simulink library "AEMS_Standard_Library"  (R2016b)
settings: Solver=ode45  StartTime=0.0  StopTime=10.0  RelTol=1e-3
undefined symbols (not defined in the file or in its folder): BkPY, carto, Cbx_extegr, Cbx_lpegrsys, Cbx_portegr, Cnx_bnk_nr_conf, Cnx_cyl_nr_conf, ConfigManagement, configuration_management, Cxx_dcm_io_tmr_end_xxxx, Cxx_dcm_rt_tmr_end, Cxx_DID_xxxx_IO_max, Cxx_DID_xxxx_IO_min, Cxx_egrhsofs, Cxx_vmaniegi, DEM_DEBOUNCE_FREEZE, DEM_DTR_CTL_INVISIBLE, DEM_DTR_CTL_NORMAL, Dem_DtrId2_XXX, Dem_DtrId3_XXX, Dem_DtrId4_XXX, Dem_DtrId5_XXX, Dem_DtrId6_XXX, Dem_DtrId7_XXX, Dem_DtrId8_XXX, Dem_DtrId9_XXX, Dem_DtrId_XXX, Dem_EnableConditionId2_XXX, Dem_EnableConditionId3_XXX, Dem_EnableConditionId4_XXX, Dem_EnableConditionId5_XXX, Dem_EnableConditionId6_XXX, Dem_EnableConditionId7_XXX, Dem_EnableConditionId8_XXX, Dem_EnableConditionId_XXX, Dem_EventId, Dem_EventId2_XXX, Dem_EventId3_XXX, Dem_EventId4_XXX, Dem_EventId5_XXX, Dem_EventId6_XXX, Dem_EventId7_XXX, Dem_EventId8_XXX, Dem_EventId9_XXX, Dem_EventId_Device_Faulttype, Dem_EventId_XXX, DEM_IUMPR_GENERAL_DENOMINATOR, DEM_OPCYC_IGNITION, Dem_RatioId2_XXX, Dem_RatioId3_XXX, Dem_RatioId4_XXX, Dem_RatioId5_XXX, Dem_RatioId6_XXX, Dem_RatioId7_XXX, Dem_RatioId8_XXX, Dem_RatioId_XXX, Dem_StorageConditionId2_XXX, Dem_StorageConditionId3_XXX, Dem_StorageConditionId4_XXX, Dem_StorageConditionId5_XXX ... (+65)
libraries: AEMS_Standard_Library x477, simulink x2
(part 16 of 39)

== system AEMS_Standard_Library/DCM/AEMS_FXP_TO_FLOAT ==
  fxp : Inport  PortDimensions=1
      settings: AttributesFormatString=<tsample=%<SampleTime>>
  Constant : Constant  Value=Resol  OutDataTypeStr=Inherit: Inherit via back propagation
  Constant1 : Constant  Value=Offset  OutDataTypeStr=Inherit: Inherit via back propagation
  Data Type Conversion : DataTypeConversion
  Product1 : Product  OutDataTypeStr=Inherit: Inherit via back propagation  SaturateOnIntegerOverflow=on  RndMeth=Zero
      settings: AttributesFormatString=SAT = %<SaturateOnIntegerOverflow>
  Sum1 : Sum  OutDataTypeStr=Inherit: Inherit via back propagation  RndMeth=Zero  SaturateOnIntegerOverflow=on  InputSameDT=on
      settings: AttributesFormatString=SAT = %<SaturateOnIntegerOverflow>
  phys : Outport
  wires:
  Data Type Conversion/1 -> Product1/1
  Constant1/1 -> Sum1/2
  Constant/1 -> Product1/2
  Sum1/1 -> phys/1
  fxp/1 -> Data Type Conversion/1
  Product1/1 -> Sum1/1

== system AEMS_Standard_Library/DCM/AEMS_RAM_SET_MAX ==
  input : Inport
      settings: AttributesFormatString=<tsample=%<SampleTime>>
  start : Inport  Port=2  OutDataTypeStr=boolean
      settings: AttributesFormatString=<tsample=%<SampleTime>>
  clear : Inport  Port=3  OutDataTypeStr=boolean
      settings: AttributesFormatString=<tsample=%<SampleTime>>
  MinMax3 : MinMax  Function=max  Inputs=2  SaturateOnIntegerOverflow=on  InputSameDT=on
  Switch1 : Switch  Threshold=0.5  SaturateOnIntegerOverflow=on  InputSameDT=on
      settings: AttributesFormatString=<threshold=%<threshold>>
  Switch5 : Switch  Threshold=0.5  SaturateOnIntegerOverflow=on  InputSameDT=on
      settings: AttributesFormatString=<threshold=%<threshold>>
  Unit Delay : UnitDelay  InitialCondition=initial_value  SampleTime=-1
      settings: AttributesFormatString=<initial=%<X0>>
  imm_const7 : Constant  Value=initial_value  OutDataTypeStr=Inherit: Inherit via back propagation
  max_value : Outport
  wires:
  input/1 -> MinMax3/1  "input"
  Switch1/1 -> Switch5/3
  clear/1 -> Switch5/2  "clear"
  MinMax3/1 -> Switch1/1  "max"
  Unit Delay/1 -> MinMax3/2, Switch1/3
  start/1 -> Switch1/2  "start"
  Switch5/1 -> max_value/1, Unit Delay/1  "max_value"
  imm_const7/1 -> Switch5/1

== system AEMS_Standard_Library/DCM/AEMS_RAM_SET_MIN ==
  input : Inport
      settings: AttributesFormatString=<tsample=%<SampleTime>>
  start : Inport  Port=2  OutDataTypeStr=boolean
      settings: AttributesFormatString=<tsample=%<SampleTime>>
  clear : Inport  Port=3  OutDataTypeStr=boolean
      settings: AttributesFormatString=<tsample=%<SampleTime>>
  MinMax3 : MinMax  Inputs=2  SaturateOnIntegerOverflow=on  InputSameDT=on
  Switch1 : Switch  Threshold=0.5  SaturateOnIntegerOverflow=on  InputSameDT=on
      settings: AttributesFormatString=<threshold=%<threshold>>
  Switch5 : Switch  Threshold=0.5  SaturateOnIntegerOverflow=on  InputSameDT=on
      settings: AttributesFormatString=<threshold=%<threshold>>
  Unit Delay : UnitDelay  InitialCondition=initial_value  SampleTime=-1
      settings: AttributesFormatString=<initial=%<X0>>
  imm_const7 : Constant  Value=initial_value  OutDataTypeStr=Inherit: Inherit via back propagation
  min_value : Outport
  wires:
  input/1 -> MinMax3/1  "input"
  Switch1/1 -> Switch5/3
  clear/1 -> Switch5/2  "clear"
  MinMax3/1 -> Switch1/1  "min"
  Unit Delay/1 -> MinMax3/2, Switch1/3
  start/1 -> Switch1/2  "start"
  Switch5/1 -> min_value/1, Unit Delay/1  "min_value"
  imm_const7/1 -> Switch5/1

== system AEMS_Standard_Library/DCM/AEMS_TO_FXP_WITH_LIMIT ==
  phys_value : Inport
  Data Type Conversion : DataTypeConversion
  Max : Constant  Value=Max  OutDataTypeStr=single
  Min : Constant  Value=Min  OutDataTypeStr=single
  MinMax : MinMax  Inputs=2  OutDataTypeStr=single  RndMeth=Zero  SaturateOnIntegerOverflow=on  InputSameDT=on
  MinMax1 : MinMax  Function=max  Inputs=2  OutDataTypeStr=single  RndMeth=Zero  SaturateOnIntegerOverflow=on  InputSameDT=on
  Offset : Constant  Value=Offset  OutDataTypeStr=single
  OutputDatatype : DataTypeConversion  OutDataTypeStr=int8  SaturateOnIntegerOverflow=on
  Product : Product  Inputs=*/  OutDataTypeStr=single  SaturateOnIntegerOverflow=on  RndMeth=Zero
      settings: AttributesFormatString=SAT = %<SaturateOnIntegerOverflow>
  Resolution : Constant  Value=Resol  OutDataTypeStr=single
  Sum : Sum  Inputs=+-  OutDataTypeStr=single  RndMeth=Zero  SaturateOnIntegerOverflow=on  InputSameDT=on
      settings: AttributesFormatString=SAT = %<SaturateOnIntegerOverflow>
  fxp_value : Outport
  wires:
  Data Type Conversion/1 -> MinMax1/1
  MinMax/1 -> Sum/1
  Resolution/1 -> Product/2
  Min/1 -> MinMax1/2
  OutputDatatype/1 -> fxp_value/1
  Sum/1 -> Product/1
  MinMax1/1 -> MinMax/2
  Max/1 -> MinMax/1
  Offset/1 -> Sum/2
  phys_value/1 -> Data Type Conversion/1
  Product/1 -> OutputDatatype/1

== system AEMS_Standard_Library/DEM/AEMS_DEM_COUNTER_BASED_DEBOUNCE ==
  flag_set : Inport
  conditionfulfilled : Inport  Port=2
  prefailed : Inport  Port=3
  prepassed : Inport  Port=4
  cleardatarequest : Inport  Port=5
  reseteventdebounce : Inport  Port=6
  AEMS_DEM_COUNTER_BASED_DEBOUNCE_D : AEMS_Standard_Library/SUB/AEMS_DEM_COUNTER_BASED_DEBOUNCE_1D  Tag=[LIB]  Description=This subsystem is interface for self diagnosis standard calculated from similar condition and NG judgment.  eventid=Dem_EventId_Device_Faulttype  DemDebounceBehavior1=DEM_DEBOUNCE_FREEZE (0)  DemCounterFailedThreshold=Cnx_dem_fail_thd_Device_Faulttype  DemCounterIncrementStepSize=Cnx_dem_pfail_inc_step_Device_Faulttype  DemCounterJumpUp=Cbx_dem_jmp_up_act_Device_Faulttype  DemCounterJumpUpValue=Cnx_dem_jmp_up_pfail_Device_Faulttype  DemCounterPassedThreshold=Cnx_dem_pass_thd_Device_Faulttype  DemCounterDecrementStepSize=Cnx_dem_ppass_dec_step_Device_Faulttype  DemCounterJumpDown=Cbx_dem_jmp_dwn_act_Device_Faulttype  DemCounterJumpDownValue=Cnx_dem_jmp_dwn_ppass_Device_Faulttype  DemCounterBypassFailure=Cbx_dem_byp_fail_Device_Faulttype
      settings: AttributesFormatString=|
      | %<MaskType>
      | EventId: %<eventid>\nDem Debounce Behavior = %<DemDebounceBehavior1>\nDem Debounce Counter Failed Threshold = %<DemCounterFailedThreshold>\nDem Debounce Counter Increment Step Size = %<DemCounterIncrementStepSize>\nDem Debounce Counter Jump Up = %<DemCounterJumpUp>\nDem Debounce Counter Jump Up Value = %<DemCounterJumpUpValue>\nDem Debounce Counter Passed Threshold = %<DemCounterPassedThreshold>\nDem Debounce Counter Decrement Step Size = %<DemCounterDecrementStepSize>\nDem Debounce Counter Jump Down = %<DemCounterJumpDown>\nDem Debounce Counter Jump Down Value = %<DemCounterJumpDownValue>\nDem Debounce Counter Bypass Failure = %<DemCounterBypassFailure>
  Logical Operator : Logic  Operator=OR  OutDataTypeStr=boolean
  debouncevalue : Outport
  failed : Outport  Port=2
  passed : Outport  Port=3
  wires:
  cleardatarequest/1 -> Logical Operator/1
  reseteventdebounce/1 -> Logical Operator/2
  Logical Operator/1 -> AEMS_DEM_COUNTER_BASED_DEBOUNCE_D/5  "reseteventdebounce"
  flag_set/1 -> AEMS_DEM_COUNTER_BASED_DEBOUNCE_D/1
  conditionfulfilled/1 -> AEMS_DEM_COUNTER_BASED_DEBOUNCE_D/2  "conditionfulfilled"
  prefailed/1 -> AEMS_DEM_COUNTER_BASED_DEBOUNCE_D/3  "prefailed"
  prepassed/1 -> AEMS_DEM_COUNTER_BASED_DEBOUNCE_D/4  "prepassed"
  AEMS_DEM_COUNTER_BASED_DEBOUNCE_D/3 -> passed/1
  AEMS_DEM_COUNTER_BASED_DEBOUNCE_D/2 -> failed/1
  AEMS_DEM_COUNTER_BASED_DEBOUNCE_D/1 -> debouncevalue/1

== system AEMS_Standard_Library/DEM/AEMS_DEM_COUNTER_BASED_DEBOUNCE_THRSHOLD_DYN ==
  flag_set : Inport
  conditionfulfilled : Inport  Port=2
  prefailed : Inport  Port=3
  prepassed : Inport  Port=4
  failedthreshold : Inport  Port=5
  passedthreshold : Inport  Port=6
  cleardatarequest : Inport  Port=7
  reseteventdebounce : Inport  Port=8
  AEMS_DEM_COUNTER_BASED_DEBOUNCE_THRSHOLD_DYN_D : AEMS_Standard_Library/SUB/AEMS_DEM_COUNTER_BASED_DEBOUNCE_THRSHOLD_DYN_1D  Tag=[LIB]  Description=This subsystem is interface for self diagnosis standard calculated from similar condition and NG judgment.  eventid=Dem_EventId_Device_Faulttype  DemDebounceBehavior1=DEM_DEBOUNCE_FREEZE (0)  DemCounterIncrementStepSize=Cnx_dem_pfail_inc_step_Device_Faulttype  DemCounterJumpUp=Cbx_dem_jmp_up_act_Device_Faulttype  DemCounterJumpUpValue=Cnx_dem_jmp_up_pfail_Device_Faulttype  DemCounterDecrementStepSize=Cnx_dem_ppass_dec_step_Device_Faulttype  DemCounterJumpDown=Cbx_dem_jmp_dwn_act_Device_Faulttype  DemCounterJumpDownValue=Cnx_dem_jmp_dwn_ppass_Device_Faulttype  DemCounterBypassFailure=Cbx_dem_byp_fail_Device_Faulttype
      settings: AttributesFormatString=|
      | %<MaskType>\nEventId: %<eventid>
      | Dem Debounce Behavior = %<DemDebounceBehavior1>
      | Dem Debounce Counter Increment Step Size = %<DemCounterIncrementStepSize>
      | Dem Debounce Counter Jump Up = %<DemCounterJumpUp>
      | Dem Debounce Counter Jump Up Value = %<DemCounterJumpUpValue>
      | Dem Debounce Counter Decrement Step Size = %<DemCounterDecrementStepSize>
      | Dem Debounce Counter Jump Down = %<DemCounterJumpDown>
      | Dem Debounce Counter Jump Down Value = %<DemCounterJumpDownValue>
      | Dem Debounce Counter Bypass Failure = %<DemCounterBypassFailure>
  AEMS_SRFLIPFLOP : AEMS_Standard_Library/FLAG/AEMS_SRFLIPFLOP  Tag=[LIB]  init=false
      settings: AttributesFormatString=%<MaskType>\nInitial condition (state of Q): = %<init>
  Data Store Write : DataStoreWrite  DataStoreName=Dem_EventId_Device_Faulttype
  Data Type Conversion : DataTypeConversion
  Logical Operator : Logic  Operator=OR  OutDataTypeStr=boolean
  debouncevalue : Outport
  failed : Outport  Port=2
  passed : Outport  Port=3
  wires:
  cleardatarequest/1 -> Logical Operator/1
  reseteventdebounce/1 -> Logical Operator/2
  Logical Operator/1 -> AEMS_DEM_COUNTER_BASED_DEBOUNCE_THRSHOLD_DYN_D/7  "reseteventdebounce"
  AEMS_DEM_COUNTER_BASED_DEBOUNCE_THRSHOLD_DYN_D/1 -> debouncevalue/1
  AEMS_DEM_COUNTER_BASED_DEBOUNCE_THRSHOLD_DYN_D/2 -> failed/1, AEMS_SRFLIPFLOP/1
  AEMS_DEM_COUNTER_BASED_DEBOUNCE_THRSHOLD_DYN_D/3 -> passed/1, AEMS_SRFLIPFLOP/2
  prepassed/1 -> AEMS_DEM_COUNTER_BASED_DEBOUNCE_THRSHOLD_DYN_D/4  "prepassed"
  prefailed/1 -> AEMS_DEM_COUNTER_BASED_DEBOUNCE_THRSHOLD_DYN_D/3  "prefailed"
  conditionfulfilled/1 -> AEMS_DEM_COUNTER_BASED_DEBOUNCE_THRSHOLD_DYN_D/2  "conditionfulfilled"
  flag_set/1 -> AEMS_DEM_COUNTER_BASED_DEBOUNCE_THRSHOLD_DYN_D/1
  failedthreshold/1 -> AEMS_DEM_COUNTER_BASED_DEBOUNCE_THRSHOLD_DYN_D/5
  passedthreshold/1 -> AEMS_DEM_COUNTER_BASED_DEBOUNCE_THRSHOLD_DYN_D/6
  AEMS_SRFLIPFLOP/1 -> Data Type Conversion/1
  Data Type Conversion/1 -> Data Store Write/1

== system AEMS_Standard_Library/DEM/AEMS_DEM_GET_EVENT_STS ==
  AEMS_DEM_GET_EVENT_STS_D : AEMS_Standard_Library/SUB/AEMS_DEM_GET_EVENT_STS_1D  Tag=[LIB]  EventId=EventId_XXXX  LibType=_DGN  FunctionMode=Dysfunctional
      settings: AttributesFormatString=%<MaskType>\nEventId : = %<EventId>\nDEM Library type : = %<LibType>\nFunction Mode : = %<FunctionMode>
  diag_status_flag : Outport
  wires:
  AEMS_DEM_GET_EVENT_STS_D/1 -> diag_status_flag/1  "diag_status_flag"

== system AEMS_Standard_Library/DEM/AEMS_DEM_GET_INDICATOR_STS ==
  AEMS_DEM_GETINDICATORSTATUS : AEMS_Standard_Library/SUB/AEMS_DEM_GETINDICATORSTATUS  Tag=[LIB]  IndicatorId=0 : IndicatorOff  SimulationMode=0 : Indicator off mode
      settings: AttributesFormatString=|
      | %<MaskType>\nIndicatorId = %<IndicatorId>
      | Simulation Mode = %<SimulationMode>
  IndicatorId_Block : Constant  Value=IndicatorOff  OutDataTypeStr=uint8
  indicator_status : Outport
  wires:
  IndicatorId_Block/1 -> AEMS_DEM_GETINDICATORSTATUS/1
  AEMS_DEM_GETINDICATORSTATUS/1 -> indicator_status/1  "indicator_status"

== system AEMS_Standard_Library/DEM/AEMS_DEM_READ_DATA_PID01 ==
  AEMS_DEM_READDATAOFPID01 : AEMS_Standard_Library/SUB/AEMS_DEM_READDATAOFPID01  Tag=[LIB]
      settings: AttributesFormatString=%<MaskType>
  vpid01 : Outport
  wires:
  AEMS_DEM_READDATAOFPID01/1 -> vpid01/1

== system AEMS_Standard_Library/DEM/AEMS_DEM_REP_IUMPR ==
  denlock_status : Inport
  faultdetect_trigger : Inport  Port=2
  DEM_REP_IUMPR_D : AEMS_Standard_Library/SUB/AEMS_DEM_REP_IUMPR_1D  Tag=[LIB]  RatioId=Dem_RatioId_XXX
      settings: AttributesFormatString=%<MaskType>\nRatioId : = %<RatioId>
  wires:
  faultdetect_trigger/1 -> DEM_REP_IUMPR_D/2  "faultdetect_trigger"
  denlock_status/1 -> DEM_REP_IUMPR_D/1  "denlock_status"

== system AEMS_Standard_Library/DEM/AEMS_DEM_REP_IUMPR_DEN_RELEASE ==
  denlock_status : Inport  OutDataTypeStr=boolean
  DEM_REP_IUMPR_DEN_RELEASE_D : AEMS_Standard_Library/SUB/AEMS_DEM_REP_IUMPR_DEN_RELEASE_1D  Tag=[LIB]  RatioId=Dem_RatioId_XXX
      settings: AttributesFormatString=%<MaskType>\nRatioId : = %<RatioId>
  wires:
  denlock_status/1 -> DEM_REP_IUMPR_DEN_RELEASE_D/1  "denlock_status"

== system AEMS_Standard_Library/DEM/AEMS_DEM_REP_IUMPR_FAULTDETECT ==
  faultdetect_trigger : Inport  OutDataTypeStr=boolean
  DEM_REP_IUMPR_FAULTDETECT_D : AEMS_Standard_Library/SUB/AEMS_DEM_REP_IUMPR_FAULTDETECT_1D  Tag=[LIB]  RatioId=Dem_RatioId_XXX
      settings: AttributesFormatString=%<MaskType>\nRatioId : = %<RatioId>
  wires:
  faultdetect_trigger/1 -> DEM_REP_IUMPR_FAULTDETECT_D/1  "faultdetect_trigger"

== system AEMS_Standard_Library/DEM/AEMS_DEM_SET_DTR ==
  set_flag : Inport  Interpolate=off
  testresult : Inport  Port=2  Interpolate=off
  lowerlimit : Inport  Port=3  Interpolate=off
  upperlimit : Inport  Port=4  Interpolate=off
  ctrl_flag : Inport  Port=5  Interpolate=off
  DEM_SET_DTR_D : AEMS_Standard_Library/SUB/AEMS_DEM_SET_DTR_1DU  Tag=[LIB]  conv_type=0x24  EventId=Dem_DtrId_XXX  resol=1  dlim=0  ulim=65535
      settings: AttributesFormatString=%<MaskType>\nConversion Type : = %<conv_type>\nEventId = %<EventId>\nresolution = %<resol>\nlowerlimit = %<dlim>\nupperlimit = %<ulim>
  wires:
  ctrl_flag/1 -> DEM_SET_DTR_D/5  "ctrl_flag"
  lowerlimit/1 -> DEM_SET_DTR_D/3  "lowerlimit"
  upperlimit/1 -> DEM_SET_DTR_D/4  "upperlimit"
  testresult/1 -> DEM_SET_DTR_D/2  "testresult"
  set_flag/1 -> DEM_SET_DTR_D/1  "set_flag"

== system AEMS_Standard_Library/DEM/AEMS_DEM_SET_ENBL_COND ==
  conditionfulfilled : Inport
  DEM_SET_ENBL_COND_D : AEMS_Standard_Library/SUB/AEMS_DEM_SET_ENBL_COND_1D  Tag=[LIB]  EnCondId=Dem_EnableConditionId_XXX
      settings: AttributesFormatString=%<MaskType>\nEnable Condition Id : = %<EnCondId>
  wires:
  conditionfulfilled/1 -> DEM_SET_ENBL_COND_D/1  "conditionfulfilled"

== system AEMS_Standard_Library/DEM/AEMS_DEM_SET_EVENT_AVL ==
  DEM_SET_EVENT_AVL_D : AEMS_Standard_Library/SUB/AEMS_DEM_SET_EVENT_AVL_1D  Tag=[LIB]  EventId=Dem_EventId  DiagROMFLAG=Diag_ROMFLAG
      settings: AttributesFormatString=%<MaskType>\nEventId = %<EventId>\nDiagROMFLAG = %<DiagROMFLAG>
  dgnsw : Outport
  wires:
  DEM_SET_EVENT_AVL_D/1 -> dgnsw/1

== system AEMS_Standard_Library/DEM/AEMS_DEM_SET_EVENT_DSBL ==
  set_flag : Inport
  DEM_SET_EVENT_DSBL_D : AEMS_Standard_Library/SUB/AEMS_DEM_SET_EVENT_DSBL_1D  Tag=[LIB]  EventId=Dem_EventId_XXX
      settings: AttributesFormatString=%<MaskType>\nEventId : = %<EventId>
  wires:
  set_flag/1 -> DEM_SET_EVENT_DSBL_D/1  "set_flag"

== system AEMS_Standard_Library/DEM/AEMS_DEM_SET_EVENT_STS ==
  diag_set_input_flag : Inport
  AEMS_DEM_SET_EVENT_STS_D : AEMS_Standard_Library/SUB/AEMS_DEM_SET_EVENT_STS_1D  Tag=[LIB]  EventId=Dem_EventId_XXX  LibType=_DGNTRP
      settings: AttributesFormatString=%<MaskType>\nEventId : = %<EventId>\nDEM Library type : = %<LibType>
  wires:
  diag_set_input_flag/1 -> AEMS_DEM_SET_EVENT_STS_D/1  "diag_set_input_flag"

== system AEMS_Standard_Library/DEM/AEMS_DEM_SET_IUMPR_DCOND ==
  condition_status : Inport
  set_flag : Inport  Port=2
  Dem_SetIUMPRDenCondition_Call : Subsystem
  wires:
  set_flag/1 -> Dem_SetIUMPRDenCondition_Call/Enable  "set_flag"
  condition_status/1 -> Dem_SetIUMPRDenCondition_Call/1(condition_status)  "condition_status"

== system AEMS_Standard_Library/DEM/AEMS_DEM_SET_OPCYC_STE ==
  cycle_state : Inport
  set_flag : Inport  Port=2
  AEMS_EDGE_RISING : AEMS_Standard_Library/EDGE/AEMS_EDGE_RISING  Tag=[LIB]  init=false
      settings: AttributesFormatString=|
      | %<MaskType>
      | Initial Value : %<init>
  Dem_SetOperationCycleState_Call : Subsystem
  wires:
  AEMS_EDGE_RISING/1 -> Dem_SetOperationCycleState_Call/Enable  "call"
  cycle_state/1 -> Dem_SetOperationCycleState_Call/1(cycle_state)  "cycle_state"
  set_flag/1 -> AEMS_EDGE_RISING/1  "set_flag"

== system AEMS_Standard_Library/DEM/AEMS_DEM_SET_PFC_CYC_QUALD ==
  set_flag : Inport
  Dem_SetPfcCycleQualified_Call : Subsystem
  wires:
  set_flag/1 -> Dem_SetPfcCycleQualified_Call/Enable  "set_flag"

== system AEMS_Standard_Library/DEM/AEMS_DEM_SET_STORAGE_COND ==
  conditionfulfilled : Inport
  DEM_SET_STORAGE_COND_D : AEMS_Standard_Library/SUB/AEMS_DEM_SET_STORAGE_COND_1D  Tag=[LIB]  StorageCondId=Dem_StorageConditionId_XXX
      settings: AttributesFormatString=%<MaskType>\nStorage Condition Id : = %<StorageCondId>
  wires:
  conditionfulfilled/1 -> DEM_SET_STORAGE_COND_D/1  "conditionfulfilled"

== system AEMS_Standard_Library/DEM/AEMS_DEM_TIME_BASED_DEBOUNCE ==
  flag_set : Inport
  conditionfulfilled : Inport  Port=2  OutDataTypeStr=boolean
  prefailed : Inport  Port=3  OutDataTypeStr=boolean
  prepassed : Inport  Port=4  OutDataTypeStr=boolean
  cleardatarequest : Inport  Port=5  OutDataTypeStr=boolean
  reseteventdebounce : Inport  Port=6  OutDataTypeStr=boolean
  AEMS_DEM_TIME_BASED_DEBOUNCE_D : AEMS_Standard_Library/SUB/AEMS_DEM_TIME_BASED_DEBOUNCE_1D  Tag=[LIB]  Description=This subsystem is interface for self diagnosis standard calculated from similar condition and NG judgment.  eventid=Dem_EventId_Device_Faulttype  DemDebounceBehavior1=DEM_DEBOUNCE_FREEZE (0)  DemDebounceTimeFailedThreshold=Cxx_dem_fail_thd_Device_Faulttype  DemDebounceTimePassedThreshold=Cxx_dem_pass_thd_Device_Faulttype  DemTimeBypassFailure=Cbx_dem_byp_fail_Device_Faulttype  Sample_Time=0.01
      settings: AttributesFormatString=|
      | %<MaskType>
      | EventId: %<eventid>\nDem Debounce Behavior = %<DemDebounceBehavior1>\nDem Debounce Time Failed Threshold = %<DemDebounceTimeFailedThreshold>\nDem Debounce Time Passed Threshold = %<DemDebounceTimePassedThreshold>\nDem Debounce Time Bypass Failure = %<DemTimeBypassFailure>\nSample_Time = %<Sample_Time>
  AEMS_SRFLIPFLOP : AEMS_Standard_Library/FLAG/AEMS_SRFLIPFLOP  Tag=[LIB]  init=false
      settings: AttributesFormatString=%<MaskType>\nInitial condition (state of Q): = %<init>
  Data Store Write : DataStoreWrite  DataStoreName=Dem_EventId_Device_Faulttype
  Data Type Conversion : DataTypeConversion
  Logical Operator : Logic  Operator=OR  OutDataTypeStr=boolean
  debouncevalue_for_failed : Outport
  debouncevalue_for_passed : Outport  Port=2
  failed : Outport  Port=3
  passed : Outport  Port=4
  wires:
  AEMS_DEM_TIME_BASED_DEBOUNCE_D/1 -> debouncevalue_for_failed/1
  AEMS_DEM_TIME_BASED_DEBOUNCE_D/2 -> debouncevalue_for_passed/1
  AEMS_DEM_TIME_BASED_DEBOUNCE_D/3 -> failed/1, AEMS_SRFLIPFLOP/1
  AEMS_DEM_TIME_BASED_DEBOUNCE_D/4 -> passed/1, AEMS_SRFLIPFLOP/2
  prepassed/1 -> AEMS_DEM_TIME_BASED_DEBOUNCE_D/4  "prepassed"
  prefailed/1 -> AEMS_DEM_TIME_BASED_DEBOUNCE_D/3  "prefailed"
  conditionfulfilled/1 -> AEMS_DEM_TIME_BASED_DEBOUNCE_D/2  "conditionfulfilled"
  flag_set/1 -> AEMS_DEM_TIME_BASED_DEBOUNCE_D/1
  Logical Operator/1 -> AEMS_DEM_TIME_BASED_DEBOUNCE_D/5  "reseteventdebounce"
  reseteventdebounce/1 -> Logical Operator/2
  cleardatarequest/1 -> Logical Operator/1
  AEMS_SRFLIPFLOP/1 -> Data Type Conversion/1
  Data Type Conversion/1 -> Data Store Write/1

== system AEMS_Standard_Library/DEM/AEMS_DEM_TIME_BASED_DEBOUNCE_THRSHOLD_DYN ==
  note: prepassed
  flag_set : Inport
  conditionfulfilled : Inport  Port=2  OutDataTypeStr=boolean
  prefailed : Inport  Port=3  OutDataTypeStr=boolean
  prepassed : Inport  Port=4  OutDataTypeStr=boolean
  cleardatarequest : Inport  Port=5  OutDataTypeStr=boolean
  reseteventdebounce : Inport  Port=6  OutDataTypeStr=boolean
  failedthreshold : Inport  Port=7
  passedthreshold : Inport  Port=8
  AEMS_DEM_TIME_BASED_DEBOUNCE_THRSHOLD_DYN_D : AEMS_Standard_Library/SUB/AEMS_DEM_TIME_BASED_DEBOUNCE_THRSHOLD_DYN_1D  Tag=[LIB]  Description=This subsystem is interface for self diagnosis standard calculated from similar condition and NG judgment.  eventid=Dem_EventId_Device_Faulttype  DemDebounceBehavior1=DEM_DEBOUNCE_FREEZE (0)  DemTimeBypassFailure=Cbx_dem_byp_fail_Device_Faulttype  Sample_Time=0.01
      settings: AttributesFormatString=|
      | %<MaskType>
      | EventId: %<eventid>\nDem Debounce Behavior = %<DemDebounceBehavior1>\nDem Debounce Time Bypass Failure = %<DemTimeBypassFailure>\nSample_Time = %<Sample_Time>
  Logical Operator : Logic  Operator=OR  OutDataTypeStr=boolean
  debouncevalue_for_failed : Outport
  debouncevalue_for_passed : Outport  Port=2
  failed : Outport  Port=3
  passed : Outport  Port=4
  wires:
  passedthreshold/1 -> AEMS_DEM_TIME_BASED_DEBOUNCE_THRSHOLD_DYN_D/7  "passedthreshold"
  failedthreshold/1 -> AEMS_DEM_TIME_BASED_DEBOUNCE_THRSHOLD_DYN_D/6  "failedthreshold"
  prefailed/1 -> AEMS_DEM_TIME_BASED_DEBOUNCE_THRSHOLD_DYN_D/3  "prefailed"
  flag_set/1 -> AEMS_DEM_TIME_BASED_DEBOUNCE_THRSHOLD_DYN_D/1
  conditionfulfilled/1 -> AEMS_DEM_TIME_BASED_DEBOUNCE_THRSHOLD_DYN_D/2  "conditionfulfilled"
  prepassed/1 -> AEMS_DEM_TIME_BASED_DEBOUNCE_THRSHOLD_DYN_D/4
  Logical Operator/1 -> AEMS_DEM_TIME_BASED_DEBOUNCE_THRSHOLD_DYN_D/5  "reseteventdebounce"
  AEMS_DEM_TIME_BASED_DEBOUNCE_THRSHOLD_DYN_D/4 -> passed/1
  AEMS_DEM_TIME_BASED_DEBOUNCE_THRSHOLD_DYN_D/3 -> failed/1
  AEMS_DEM_TIME_BASED_DEBOUNCE_THRSHOLD_DYN_D/2 -> debouncevalue_for_passed/1
  AEMS_DEM_TIME_BASED_DEBOUNCE_THRSHOLD_DYN_D/1 -> debouncevalue_for_failed/1
  reseteventdebounce/1 -> Logical Operator/2
  cleardatarequest/1 -> Logical Operator/1

== system AEMS_Standard_Library/DEM/AEMS_FIM_GETFUNCTIONINHIBITION ==
  AEMS_FIM_GET_FUNC_PMT_D : AEMS_Standard_Library/SUB/AEMS_FIM_GET_FUNC_PMT_1D  Tag=[LIB]  FID=Fim_fid_xxxx  FunctionMode=Functional
      settings: AttributesFormatString=%<MaskType>\nFunction Mode = %<FunctionMode>\nDowngraded mode short name : = %<FID>
  InhibitionStatus : Outport
  wires:
  AEMS_FIM_GET_FUNC_PMT_D/1 -> InhibitionStatus/1  "InhibitionStatus"

== system AEMS_Standard_Library/DISCONTINUITIES/AEMS_DEADZONE ==
  input_signal : Inport
  start_end_zone : Inport  Port=2
  end_dead_zone : Inport  Port=3
  Constant1 : Constant  Value=mf  OutDataTypeStr=Inherit: Inherit via back propagation
  Product : Product  OutDataTypeStr=Inherit: Inherit via back propagation  RndMeth=Zero
  RelationalOperator2 : RelationalOperator  Operator=>  OutDataTypeStr=boolean  RndMeth=Nearest  InputSameDT=on
  RelationalOperator3 : RelationalOperator  Operator=<  OutDataTypeStr=boolean  RndMeth=Nearest  InputSameDT=on
  Sum{,1..3} (4 alike) : Sum  Inputs=+-  OutDataTypeStr=Inherit: Inherit via back propagation  RndMeth=Zero  InputSameDT=on
  Switch1 : Switch  Criteria=u2 ~= 0  RndMeth=Zero  SaturateOnIntegerOverflow=on  InputSameDT=on
      settings: AttributesFormatString=Criteria=%<Criteria>
  Switch4 : Switch  Criteria=u2 ~= 0  RndMeth=Zero  SaturateOnIntegerOverflow=on  InputSameDT=on
      settings: AttributesFormatString=Criteria=%<Criteria>
  UnitDelay1 : UnitDelay  SampleTime=-1
      settings: AttributesFormatString=<initial=%<InitialCondition>>
  dead_zone : Outport
  wires:
  start_end_zone/1 -> Sum/2, RelationalOperator2/1
  Switch4/1 -> UnitDelay1/1, dead_zone/1
  RelationalOperator3/1 -> Switch1/2
  RelationalOperator2/1 -> Switch4/2
  Sum3/1 -> Switch1/1
  Switch1/1 -> Switch4/3
  input_signal/1 -> Sum/1, Sum2/1, Sum3/1, Sum1/1
  Sum/1 -> Switch4/1
  end_dead_zone/1 -> RelationalOperator3/1, Sum3/2
  Product/1 -> Switch1/3, Sum1/2, Sum2/2
  UnitDelay1/1 -> Product/1
  Constant1/1 -> Product/2
  Sum1/1 -> RelationalOperator2/2
  Sum2/1 -> RelationalOperator3/2

== system AEMS_Standard_Library/DISCONTINUITIES/AEMS_ENUMERATION_SWITCH ==
  Control_Input : Inport
  Dataport1 : Inport  Port=2
  Dataport2 : Inport  Port=3
  Dataport3 : Inport  Port=4
  MultiportSwitch : MultiPortSwitch  DataPortOrder=Specify indices  Inputs=2  DataPortIndices={[Nnx_aaa_stt,Nnx_bbb_stt],Nnx_ccc_stt,Nnx_ddd_stt}  DiagnosticForDefault=None
  Out : Outport
  wires:
  Dataport2/1 -> MultiportSwitch/3
  Dataport1/1 -> MultiportSwitch/2
  MultiportSwitch/1 -> Out/1
  Control_Input/1 -> MultiportSwitch/1
  Dataport3/1 -> MultiportSwitch/4

== system AEMS_Standard_Library/DISCONTINUITIES/AEMS_MULTI_PORT_TIME_SWITCH ==
  Vxx_swi_t : Inport  Tag=AM,In,0,1,Name,C;CMP,Port,PortWidth,SampleTime;
  Vsx_sel : Inport  Tag=AM,In,0,1,Name,C;CMP,Port,PortWidth,SampleTime;  Port=2
  Vxx_in1 : Inport  Tag=AM,In,0,1,Name,C;CMP,Port,PortWidth,SampleTime;  Port=3
  Vxx_in2 : Inport  Tag=AM,In,0,1,Name,C;CMP,Port,PortWidth,SampleTime;  Port=4
  Vxx_in3 : Inport  Tag=AM,In,0,1,Name,C;CMP,Port,PortWidth,SampleTime;  Port=5
  Vxx_in4 : Inport  Tag=AM,In,0,1,Name,C;CMP,Port,PortWidth,SampleTime;  Port=6
  Vxx_in5 : Inport  Tag=AM,In,0,1,Name,C;CMP,Port,PortWidth,SampleTime;  Port=7
  Vxx_in6 : Inport  Tag=AM,In,0,1,Name,C;CMP,Port,PortWidth,SampleTime;  Port=8
  Vxx_in7 : Inport  Tag=AM,In,0,1,Name,C;CMP,Port,PortWidth,SampleTime;  Port=9
  Vxx_in8 : Inport  Tag=AM,In,0,1,Name,C;CMP,Port,PortWidth,SampleTime;  Port=10
  dT : Inport  Tag=AM,In,0,1,Name,C;CMP,Port,PortWidth,SampleTime;  Port=11
  Saturation : Saturate  UpperLimit=8  LowerLimit=1  RndMeth=Zero
      settings: AttributesFormatString=L_Limit = %<LowerLimit>\nU_Limit = %<UpperLimit>
  in_clc : Subsystem
  interpolation : Subsystem
  number_1_2 : Subsystem
  pulse_and_old : Subsystem
  slop_on : Subsystem
  transient_timer : Subsystem
  Vxx_out : Outport  Tag=AM,Out,1,0,Name,NC;CMP,Port,OutputWhenDisabled,InitialOutput;
  Vbx_slop_on : Outport  Tag=AM,Out,1,0,Name,NC;CMP,Port,OutputWhenDisabled,InitialOutput;  Port=2
  wires:
  Saturation/1 -> in_clc/4(Vsx_sel), pulse_and_old/1(Vsx_sel)
  dT/1 -> transient_timer/3(dT)
  in_clc/2(Vxx_out_sel_old) -> interpolation/4(Vxx_out_sel_old)
  in_clc/1(Vxx_out_sel) -> interpolation/3(Vxx_out_sel)
  slop_on/1(Vbx_slop_on) -> number_1_2/1(Vbx_slop_on), interpolation/2(Vbx_slop_on), Vbx_slop_on/1
  Vxx_in8/1 -> in_clc/12(Vxx_in8)
  Vxx_in7/1 -> in_clc/11(Vxx_in7)
  Vxx_in5/1 -> in_clc/9(Vxx_in5)
  Vxx_in6/1 -> in_clc/10(Vxx_in6)
  transient_timer/1(Vxx_swi_trs) -> interpolation/1(Vxx_swi_trs), slop_on/1(Vxx_swi_trs)
  number_1_2/1(Vsx_swi_nr) -> in_clc/1(Vsx_swi_nr)
  pulse_and_old/2(Vsx_sel_old) -> in_clc/3(Vsx_sel_old)
  Vxx_swi_t/1 -> transient_timer/1(Vxx_swi_t)
  Vsx_sel/1 -> Saturation/1
  Vxx_in4/1 -> in_clc/8(Vxx_in4)
  Vxx_in3/1 -> in_clc/7(Vxx_in3)
  Vxx_in2/1 -> in_clc/6(Vxx_in2)
  Vxx_in1/1 -> in_clc/5(Vxx_in1)
  interpolation/1(Vxx_out) -> Vxx_out/1
  pulse_and_old/1(Vbx_sel_puls) -> transient_timer/2(Vbx_sel_puls), in_clc/2(Vbx_sel_puls), number_1_2/2(Vbx_sel_puls), slop_on/2(Vbx_sel_puls)

== system AEMS_Standard_Library/DISCONTINUITIES/AEMS_SLEW_RATE ==
  Pos_Slope : Inport
  Input : Inport  Port=2
  Neg_Slope : Inport  Port=3
  Timestep : Inport  Port=4
  Product2 : Product  Tag=AM,Std,Inputs,1;CMP,Inputs;  Inputs=**  OutDataTypeStr=Inherit: Inherit via back propagation  RndMeth=Zero
      settings: AttributesFormatString=SAT = %<SaturateOnIntegerOverflow>
  Product3 : Product  Tag=AM,Std,Inputs,1;CMP,Inputs;  Inputs=**  OutDataTypeStr=Inherit: Inherit via back propagation  RndMeth=Zero
      settings: AttributesFormatString=SAT = %<SaturateOnIntegerOverflow>
  Slew_rate : Subsystem
  Output : Outport
  wires:
  Slew_rate/1(OUTPUT) -> Output/1
  Timestep/1 -> Product2/2, Product3/1
  Neg_Slope/1 -> Product3/2
  Pos_Slope/1 -> Product2/1
  Product2/1 -> Slew_rate/1(MAX_SLEW_RATE)  "MAX_SLEW_RATE"
  Product3/1 -> Slew_rate/3(MIN_SLEW_RATE)  "MIN_SLEW_RATE"
  Input/1 -> Slew_rate/2(INPUT)

== system AEMS_Standard_Library/DISCONTINUITIES/AEMS_SLOPE_SWITCH ==
  Switch_Cmd : Inport
  Pos_Slope : Inport  Port=2
  Neg_Slope : Inport  Port=3
  In0 : Inport  Port=4
  In1 : Inport  Port=5
  dT : Inport  Tag=AM,In,0,1,Name,C;CMP,Port,PortWidth,SampleTime;  Port=6
  Multiport_Switch : MultiPortSwitch  DataPortOrder=Zero-based contiguous  Inputs=2  zeroidx=on  RndMeth=Zero  SaturateOnIntegerOverflow=on  InputSameDT=on
      settings: AttributesFormatString=PortOrder=%<DataPortOrder>
  Product : Product  OutDataTypeStr=Inherit: Inherit via back propagation  SaturateOnIntegerOverflow=on  RndMeth=Zero
      settings: AttributesFormatString=SAT = %<SaturateOnIntegerOverflow>
  Product1 : Product  OutDataTypeStr=Inherit: Inherit via back propagation  SaturateOnIntegerOverflow=on  RndMeth=Zero
      settings: AttributesFormatString=SAT = %<SaturateOnIntegerOverflow>
  Signal_Change_Compute : Subsystem
  Slope_On_Block : Subsystem
  Slope_On_Compute : Subsystem
  Switch2 : Switch  Tag=GEN,Threshold;AM,Switch,2,1;CMP,Threshold;  Criteria=u2 ~= 0  RndMeth=Zero  SaturateOnIntegerOverflow=on  InputSameDT=on
      settings: AttributesFormatString=Criteria=%<Criteria>
  UnitDelay1 : UnitDelay  SampleTime=-1
      settings: AttributesFormatString=IC = %<X0>
  UnitDelay2 : UnitDelay  SampleTime=-1
      settings: AttributesFormatString=IC = %<X0>
  Output : Outport  Tag=AM,Out,1,0,Name,NC;CMP,Port,OutputWhenDisabled,InitialOutput;
  Slope_On : Outport  Tag=AM,Out,1,0,Name,NC;CMP,Port,OutputWhenDisabled,InitialOutput;  Port=2
  wires:
  dT/1 -> Product1/1, Product/2
  Neg_Slope/1 -> Product1/2
  Slope_On_Block/1(Output_Not_Equals_Input) -> UnitDelay1/1
  Multiport_Switch/1 -> Slope_On_Block/2(Input), Switch2/3  "Slope_Off"
  Signal_Change_Compute/1(Signal_Change) -> Slope_On_Block/1(Signal_Change), Slope_On_Compute/1(Signal_Change)
  Pos_Slope/1 -> Product/1
  Product1/1 -> Slope_On_Block/4(Neg_Slope)
  Product/1 -> Slope_On_Block/3(Pos_Slope)
  UnitDelay2/1 -> Slope_On_Block/5(Prev_Output)
  Switch_Cmd/1 -> Signal_Change_Compute/1(Switch_Cmd), Multiport_Switch/1
  UnitDelay1/1 -> Slope_On_Compute/2(Output_Not_Equals_Input)
  Switch2/1 -> Output/1, UnitDelay2/1
  Slope_On_Block/2(Output) -> Switch2/1
  Slope_On_Compute/1(Slope_On) -> Switch2/2, Slope_On_Block/Enable, Slope_On/1
  In0/1 -> Multiport_Switch/2
  In1/1 -> Multiport_Switch/3

== system AEMS_Standard_Library/DISCONTINUITIES/AEMS_SLOPE_SWITCH_3INPUTS ==
  Switch_Cmd : Inport  Tag=AM,In,0,1,Name,C;CMP,Port,PortWidth,SampleTime;
  Pos_Slope : Inport  Port=2
  Neg_Slope : Inport  Port=3
  In0 : Inport  Port=4
  In1 : Inport  Port=5
  In2 : Inport  Port=6
  dT : Inport  Tag=AM,In,0,1,Name,C;CMP,Port,PortWidth,SampleTime;  Port=7
  Multiport_Switch : MultiPortSwitch  DataPortOrder=Zero-based contiguous  zeroidx=on  RndMeth=Zero  SaturateOnIntegerOverflow=on  InputSameDT=on
      settings: AttributesFormatString=PortOrder=%<DataPortOrder>
  Product : Product  OutDataTypeStr=Inherit: Inherit via back propagation  SaturateOnIntegerOverflow=on  RndMeth=Zero
      settings: AttributesFormatString=SAT = %<SaturateOnIntegerOverflow>
  Product1 : Product  OutDataTypeStr=Inherit: Inherit via back propagation  SaturateOnIntegerOverflow=on  RndMeth=Zero
      settings: AttributesFormatString=SAT = %<SaturateOnIntegerOverflow>
  Signal_Change_Compute : Subsystem
  Slope_On_Block : Subsystem
  Slope_On_Compute : Subsystem
  Switch2 : Switch  Tag=GEN,Threshold;AM,Switch,2,1;CMP,Threshold;  Criteria=u2 ~= 0  RndMeth=Zero  SaturateOnIntegerOverflow=on  InputSameDT=on
      settings: AttributesFormatString=Criteria=%<Criteria>
  UnitDelay1 : UnitDelay  SampleTime=-1
      settings: AttributesFormatString=IC = %<X0>
  UnitDelay2 : UnitDelay  SampleTime=-1
      settings: AttributesFormatString=IC = %<X0>
  Output : Outport  Tag=AM,Out,1,0,Name,NC;CMP,Port,OutputWhenDisabled,InitialOutput;
  Slope_On : Outport  Tag=AM,Out,1,0,Name,NC;CMP,Port,OutputWhenDisabled,InitialOutput;  Port=2
  wires:
  Switch_Cmd/1 -> Multiport_Switch/1, Signal_Change_Compute/1(Switch_Cmd)
  In0/1 -> Multiport_Switch/2
  In1/1 -> Multiport_Switch/3
  In2/1 -> Multiport_Switch/4
  Slope_On_Compute/1(Slope_On) -> Slope_On/1, Switch2/2, Slope_On_Block/Enable  "Enable_Slope_On_Block"
  Slope_On_Block/2(Output) -> Switch2/1
  Switch2/1 -> Output/1, UnitDelay2/1
  UnitDelay1/1 -> Slope_On_Compute/2(Output_Not_Equals_Input)
  UnitDelay2/1 -> Slope_On_Block/5(Prev_Output)
  Product/1 -> Slope_On_Block/3(Pos_Slope)
  Product1/1 -> Slope_On_Block/4(Neg_Slope)
  Pos_Slope/1 -> Product/1
  Neg_Slope/1 -> Product1/1
  Signal_Change_Compute/1(Signal_Change) -> Slope_On_Compute/1(Signal_Change), Slope_On_Block/1(Signal_Change)
  Multiport_Switch/1 -> Slope_On_Block/2(Input), Switch2/3  "Slope_Off"
  dT/1 -> Product/2, Product1/2
  Slope_On_Block/1(Output_Not_Equals_Input) -> UnitDelay1/1

== system AEMS_Standard_Library/DISCONTINUITIES/AEMS_SLOPE_SWITCH_4INPUTS ==
  Switch_Cmd : Inport  Tag=AM,In,0,1,Name,C;CMP,Port,PortWidth,SampleTime;
  Pos_Slope : Inport  Port=2
  Neg_Slope : Inport  Port=3
  In0 : Inport  Port=4
  In1 : Inport  Port=5
  In2 : Inport  Port=6
  In3 : Inport  Port=7
  dT : Inport  Tag=AM,In,0,1,Name,C;CMP,Port,PortWidth,SampleTime;  Port=8
  Multiport_Switch : MultiPortSwitch  DataPortOrder=Zero-based contiguous  Inputs=4  zeroidx=on  RndMeth=Zero  SaturateOnIntegerOverflow=on  InputSameDT=on
      settings: AttributesFormatString=PortOrder=%<DataPortOrder>
  Product : Product  OutDataTypeStr=Inherit: Inherit via back propagation  SaturateOnIntegerOverflow=on  RndMeth=Zero
      settings: AttributesFormatString=SAT = %<SaturateOnIntegerOverflow>
  Product1 : Product  OutDataTypeStr=Inherit: Inherit via back propagation  SaturateOnIntegerOverflow=on  RndMeth=Zero
      settings: AttributesFormatString=SAT = %<SaturateOnIntegerOverflow>
  Signal_Change_Compute : Subsystem
  Slope_On_Block : Subsystem
  Slope_On_Compute : Subsystem
  Switch2 : Switch  Tag=GEN,Threshold;AM,Switch,2,1;CMP,Threshold;  Criteria=u2 ~= 0  RndMeth=Zero  SaturateOnIntegerOverflow=on  InputSameDT=on
      settings: AttributesFormatString=Criteria=%<Criteria>
  UnitDelay1 : UnitDelay  SampleTime=-1
      settings: AttributesFormatString=IC = %<X0>
  UnitDelay2 : UnitDelay  SampleTime=-1
      settings: AttributesFormatString=IC = %<X0>
  Output : Outport  Tag=AM,Out,1,0,Name,NC;CMP,Port,OutputWhenDisabled,InitialOutput;
  Slope_On : Outport  Tag=AM,Out,1,0,Name,NC;CMP,Port,OutputWhenDisabled,InitialOutput;  Port=2
  wires:
  Switch_Cmd/1 -> Multiport_Switch/1, Signal_Change_Compute/1(Switch_Cmd)
  In0/1 -> Multiport_Switch/2
  In1/1 -> Multiport_Switch/3
  In2/1 -> Multiport_Switch/4
  In3/1 -> Multiport_Switch/5
  Slope_On_Compute/1(Slope_On) -> Slope_On/1, Switch2/2, Slope_On_Block/Enable  "Enable_Slope_On_Block"
  Slope_On_Block/2(Output) -> Switch2/1
  Switch2/1 -> Output/1, UnitDelay2/1
  UnitDelay1/1 -> Slope_On_Compute/2(Output_Not_Equals_Input)
  UnitDelay2/1 -> Slope_On_Block/5(Prev_Output)
  Product/1 -> Slope_On_Block/3(Pos_Slope)
  Product1/1 -> Slope_On_Block/4(Neg_Slope)
  Pos_Slope/1 -> Product/1
  Neg_Slope/1 -> Product1/1
  Signal_Change_Compute/1(Signal_Change) -> Slope_On_Compute/1(Signal_Change), Slope_On_Block/1(Signal_Change)
  Multiport_Switch/1 -> Slope_On_Block/2(Input), Switch2/3  "Slope_Off"
  dT/1 -> Product/2, Product1/2
  Slope_On_Block/1(Output_Not_Equals_Input) -> UnitDelay1/1

== system AEMS_Standard_Library/DISCONTINUITIES/AEMS_SLOPE_SWITCH_6INPUTS ==
  Switch_Cmd : Inport  Tag=AM,In,0,1,Name,C;CMP,Port,PortWidth,SampleTime;
  Pos_Slope : Inport  Port=2
  Neg_Slope : Inport  Port=3
  In0 : Inport  Port=4
  In1 : Inport  Port=5
  In2 : Inport  Port=6
  In3 : Inport  Port=7
  In4 : Inport  Port=8
  In5 : Inport  Port=9
  dT : Inport  Tag=AM,In,0,1,Name,C;CMP,Port,PortWidth,SampleTime;  Port=10
  Multiport_Switch : MultiPortSwitch  DataPortOrder=Zero-based contiguous  Inputs=6  zeroidx=on  RndMeth=Zero  SaturateOnIntegerOverflow=on  InputSameDT=on
      settings: AttributesFormatString=PortOrder=%<DataPortOrder>
  Product : Product  OutDataTypeStr=Inherit: Inherit via back propagation  SaturateOnIntegerOverflow=on  RndMeth=Zero
      settings: AttributesFormatString=SAT = %<SaturateOnIntegerOverflow>
  Product1 : Product  OutDataTypeStr=Inherit: Inherit via back propagation  SaturateOnIntegerOverflow=on  RndMeth=Zero
      settings: AttributesFormatString=SAT = %<SaturateOnIntegerOverflow>
  Signal_Change_Compute : Subsystem
  Slope_On_Block : Subsystem
  Slope_On_Compute : Subsystem
  Switch2 : Switch  Tag=GEN,Threshold;AM,Switch,2,1;CMP,Threshold;  Criteria=u2 ~= 0  RndMeth=Zero  SaturateOnIntegerOverflow=on  InputSameDT=on
      settings: AttributesFormatString=Criteria=%<Criteria>
  Unit_Delay1 : UnitDelay  SampleTime=-1
      settings: AttributesFormatString=IC = %<X0>
  Unit_Delay2 : UnitDelay  SampleTime=-1
      settings: AttributesFormatString=IC = %<X0>
  Output : Outport  Tag=AM,Out,1,0,Name,NC;CMP,Port,OutputWhenDisabled,InitialOutput;
  Slope_On : Outport  Tag=AM,Out,1,0,Name,NC;CMP,Port,OutputWhenDisabled,InitialOutput;  Port=2
  wires:
  Pos_Slope/1 -> Product/1
  Neg_Slope/1 -> Product1/1
  Slope_On_Block/1(Output_Not_Equals_Input) -> Unit_Delay1/1
  dT/1 -> Product1/2, Product/2
  Multiport_Switch/1 -> Slope_On_Block/2(Input), Switch2/3
  Signal_Change_Compute/1(Signal_Change) -> Slope_On_Block/1(Signal_Change), Slope_On_Compute/1(Signal_Change)
  Product1/1 -> Slope_On_Block/4(Neg_Slope)
  Product/1 -> Slope_On_Block/3(Pos_Slope)
  Unit_Delay2/1 -> Slope_On_Block/5(Prev_Output)
  Unit_Delay1/1 -> Slope_On_Compute/2(Output_Not_Equals_Input)
  Switch2/1 -> Unit_Delay2/1, Output/1
  Slope_On_Block/2(Output) -> Switch2/1
  Slope_On_Compute/1(Slope_On) -> Slope_On_Block/Enable, Switch2/2, Slope_On/1  "Enable_Slope_On_Block"
  Switch_Cmd/1 -> Signal_Change_Compute/1(Switch_Cmd), Multiport_Switch/1
  In0/1 -> Multiport_Switch/2
  In1/1 -> Multiport_Switch/3
  In2/1 -> Multiport_Switch/4
  In3/1 -> Multiport_Switch/5
  In4/1 -> Multiport_Switch/6
  In5/1 -> Multiport_Switch/7

== system AEMS_Standard_Library/DISCONTINUITIES/AEMS_SLOPE_SWITCH_8INPUTS ==
  Switch_Cmd : Inport  Tag=AM,In,0,1,Name,C;CMP,Port,PortWidth,SampleTime;
  Pos_Slope : Inport  Port=2
  Neg_Slope : Inport  Port=3
  In0 : Inport  Port=4
  In1 : Inport  Port=5
  In2 : Inport  Port=6
  In3 : Inport  Port=7
  In4 : Inport  Port=8
  In5 : Inport  Port=9
  In6 : Inport  Port=10
  In7 : Inport  Port=11
  dT : Inport  Tag=AM,In,0,1,Name,C;CMP,Port,PortWidth,SampleTime;  Port=12
  Multiport_Switch : MultiPortSwitch  DataPortOrder=Zero-based contiguous  Inputs=8  zeroidx=on  RndMeth=Zero  SaturateOnIntegerOverflow=on  InputSameDT=on
      settings: AttributesFormatString=PortOrder=%<DataPortOrder>
  Product : Product  OutDataTypeStr=Inherit: Inherit via back propagation  SaturateOnIntegerOverflow=on  RndMeth=Zero
      settings: AttributesFormatString=SAT = %<SaturateOnIntegerOverflow>
  Product1 : Product  OutDataTypeStr=Inherit: Inherit via back propagation  SaturateOnIntegerOverflow=on  RndMeth=Zero
      settings: AttributesFormatString=SAT = %<SaturateOnIntegerOverflow>
  Signal_Change_Compute : Subsystem
  Slope_On_Block : Subsystem
  Slope_On_Compute : Subsystem
  Switch2 : Switch  Tag=GEN,Threshold;AM,Switch,2,1;CMP,Threshold;  Criteria=u2 ~= 0  RndMeth=Zero  SaturateOnIntegerOverflow=on  InputSameDT=on
      settings: AttributesFormatString=Criteria=%<Criteria>
  Unit_Delay1 : UnitDelay  SampleTime=-1
      settings: AttributesFormatString=IC = %<X0>
  Unit_Delay2 : UnitDelay  SampleTime=-1
      settings: AttributesFormatString=IC = %<X0>
  Output : Outport  Tag=AM,Out,1,0,Name,NC;CMP,Port,OutputWhenDisabled,InitialOutput;
  Slope_On : Outport  Tag=AM,Out,1,0,Name,NC;CMP,Port,OutputWhenDisabled,InitialOutput;  Port=2
  wires:
  Pos_Slope/1 -> Product/1
  Neg_Slope/1 -> Product1/1
  Slope_On_Block/1(Output_Not_Equals_Input) -> Unit_Delay1/1
  dT/1 -> Product1/2, Product/2
  Multiport_Switch/1 -> Slope_On_Block/2(Input), Switch2/3
  Signal_Change_Compute/1(Signal_Change) -> Slope_On_Block/1(Signal_Change), Slope_On_Compute/1(Signal_Change)
  Product1/1 -> Slope_On_Block/4(Neg_Slope)
  Product/1 -> Slope_On_Block/3(Pos_Slope)
  Unit_Delay2/1 -> Slope_On_Block/5(Prev_Output)
  Unit_Delay1/1 -> Slope_On_Compute/2(Output_Not_Equals_Input)
  Switch2/1 -> Unit_Delay2/1, Output/1
  Slope_On_Block/2(Output) -> Switch2/1
  Slope_On_Compute/1(Slope_On) -> Slope_On_Block/Enable, Switch2/2, Slope_On/1  "Enable_Slope_On_Block"
  Switch_Cmd/1 -> Signal_Change_Compute/1(Switch_Cmd), Multiport_Switch/1
  In0/1 -> Multiport_Switch/2
  In1/1 -> Multiport_Switch/3
  In2/1 -> Multiport_Switch/4
  In3/1 -> Multiport_Switch/5
  In4/1 -> Multiport_Switch/6
  In5/1 -> Multiport_Switch/7
  In6/1 -> Multiport_Switch/8
  In7/1 -> Multiport_Switch/9

== system AEMS_Standard_Library/DISCRETE/AEMS_UNITDELAY_EXTERNALIC ==
  u : Inport
  IC : Inport  Port=2
  FixPt_Constant1 : Constant  Value=true
  FixPt_UnitDelay1 : UnitDelay  SampleTime=-1
      settings: AttributesFormatString=IC = %<X0>
  FixPt_UnitDelay3 : UnitDelay  SampleTime=-1
      settings: AttributesFormatString=IC = %<X0>
  Init : Switch  Criteria=u2 ~= 0  RndMeth=Zero  ZeroCross=off  InputSameDT=on
      settings: AttributesFormatString=Criteria=%<Criteria>
  y : Outport
  wires:
  FixPt_UnitDelay1/1 -> Init/1
  IC/1 -> Init/3
  u/1 -> FixPt_UnitDelay1/1
  FixPt_Constant1/1 -> FixPt_UnitDelay3/1
  FixPt_UnitDelay3/1 -> Init/2
  Init/1 -> y/1

== system AEMS_Standard_Library/DISCRETE/AEMS_UNITDELAY_RESET_EXTERNALIC ==
  u : Inport
  R : Inport  Port=2
  IC : Inport  Port=3
  FixPt_Constant : Constant  DisableCoverage=on  Value=true
  FixPt_Logical_Operator : Logic  DisableCoverage=on  Operator=OR  OutDataTypeStr=boolean
  FixPt_Logical_Operator1 : Logic  DisableCoverage=on  Operator=NOT  OutDataTypeStr=boolean
  FixPt_Unit_Delay1 : UnitDelay  DisableCoverage=on  SampleTime=-1
      settings: AttributesFormatString=<initial=%<InitialCondition>>
  FixPt_Unit_Delay2 : UnitDelay  DisableCoverage=on  InitialCondition=false  SampleTime=-1
      settings: AttributesFormatString=<initial=%<InitialCondition>>
  Init : Switch  Criteria=u2 ~= 0  RndMeth=Zero  ZeroCross=off  InputSameDT=on
      settings: AttributesFormatString=Criteria=%<Criteria>
  Reset : Switch  Criteria=u2 ~= 0  RndMeth=Zero  ZeroCross=off  InputSameDT=on
      settings: AttributesFormatString=Criteria=%<Criteria>
  y : Outport
  wires:
  FixPt_Logical_Operator1/1 -> FixPt_Logical_Operator/2
  FixPt_Logical_Operator/1 -> Init/2
  Init/1 -> y/1
  FixPt_Unit_Delay2/1 -> FixPt_Logical_Operator1/1
  FixPt_Constant/1 -> FixPt_Unit_Delay2/1
  R/1 -> Reset/2, FixPt_Logical_Operator/1
  Reset/1 -> FixPt_Unit_Delay1/1  "Xnew"
  u/1 -> Reset/3
  IC/1 -> Init/1, Reset/1
  FixPt_Unit_Delay1/1 -> Init/3  "Xold"

== system AEMS_Standard_Library/EDGE/AEMS_EDGE_EITHER ==
  In : Inport
  FixPt_UnitDelay1 : UnitDelay  InitialCondition=InitValue  SampleTime=-1
      settings: AttributesFormatString=IC = %<X0>
  Logical_Operator4 : Logic  Operator=XOR  OutDataTypeStr=boolean
  Out : Outport
  wires:
  In/1 -> Logical_Operator4/1, FixPt_UnitDelay1/1
  FixPt_UnitDelay1/1 -> Logical_Operator4/2
  Logical_Operator4/1 -> Out/1

== system AEMS_Standard_Library/EDGE/AEMS_EDGE_FALLING ==
  In : Inport
  FixPt_UnitDelay1 : UnitDelay  InitialCondition=InitValue  SampleTime=-1
      settings: AttributesFormatString=IC = %<X0>
  Logical_Operator2 : Logic  OutDataTypeStr=boolean
  Logical_Operator3 : Logic  Operator=NOT  OutDataTypeStr=boolean
  Out : Outport
  wires:
  In/1 -> Logical_Operator3/1, FixPt_UnitDelay1/1
  Logical_Operator3/1 -> Logical_Operator2/1
  Logical_Operator2/1 -> Out/1  "Falling"
  FixPt_UnitDelay1/1 -> Logical_Operator2/2

== system AEMS_Standard_Library/EDGE/AEMS_EDGE_RISING ==
  In : Inport
  FixPt_UnitDelay1 : UnitDelay  InitialCondition=InitValue  SampleTime=-1
      settings: AttributesFormatString=IC = %<X0>
  Logical_Operator : Logic  OutDataTypeStr=boolean
  Logical_Operator1 : Logic  Operator=NOT  OutDataTypeStr=boolean
  Out : Outport
  wires:
  In/1 -> Logical_Operator/1, FixPt_UnitDelay1/1
  Logical_Operator1/1 -> Logical_Operator/2
  Logical_Operator/1 -> Out/1  "Rising"
  FixPt_UnitDelay1/1 -> Logical_Operator1/1

== system AEMS_Standard_Library/FILTER/AEMS_DISCRETE_TIME_INTEGRATOR_EULER ==
  note: Forward Euler: y(n) = x(n-1)*T*K + y(n-1)
  note: External reset: "rising"
  value : Inport
  trig : Inport  Port=2
  dT : Inport  Port=3
  Add1 : Sum  OutDataTypeStr=Inherit: Inherit via back propagation  RndMeth=Zero  InputSameDT=on
  Constant3 : Constant  Value=0  OutDataTypeStr=Inherit: Inherit via back propagation
  LogicalOperator : Logic  OutDataTypeStr=boolean
  LogicalOperator1 : Logic  Operator=NOT  Inputs=1  OutDataTypeStr=boolean
  Product1 : Product  OutDataTypeStr=Inherit: Inherit via back propagation  RndMeth=Zero
  Saturation : Saturate  UpperLimit=Upper_limit  LowerLimit=Lower_limit  RndMeth=Zero
      settings: AttributesFormatString=L_Limit = %<LowerLimit>\nU_Limit = %<UpperLimit>
  Switch1 : Switch  Criteria=u2 ~= 0  RndMeth=Zero  InputSameDT=on
      settings: AttributesFormatString=Criteria=%<Criteria>
  UnitDelay1 : UnitDelay  InitialCondition=false  SampleTime=-1
      settings: AttributesFormatString=IC = %<X0>
  UnitDelay2 : UnitDelay  SampleTime=-1
      settings: AttributesFormatString=IC = %<X0>
  UnitDelay3 : UnitDelay  SampleTime=-1
      settings: AttributesFormatString=IC = %<X0>
  Integrator_output : Outport
  wires:
  UnitDelay2/1 -> Product1/1
  dT/1 -> Product1/2
  value/1 -> UnitDelay2/1
  UnitDelay1/1 -> LogicalOperator/2
  trig/1 -> LogicalOperator/1, LogicalOperator1/1
  LogicalOperator1/1 -> UnitDelay1/1
  UnitDelay3/1 -> Add1/2
  Add1/1 -> Switch1/3
  LogicalOperator/1 -> Switch1/2
  Switch1/1 -> Saturation/1
  Constant3/1 -> Switch1/1
  Saturation/1 -> Integrator_output/1, UnitDelay3/1
  Product1/1 -> Add1/1
